simulink model "template_examples"  (R2024b)
settings: Solver=FixedStepDiscrete  StartTime=0.0  StopTime=10.0  RelTol=1e-3
libraries: hdlsllib x25, simulink x2
settings Model: Creator=foregan  LastModifiedBy=foregan
settings OptimizationCC: BlockReduction=off  ConditionallyExecuteInputs=off  DefaultParameterBehavior=Inlined
settings DebuggingCC: AlgebraicLoopMsg=error  SingleTaskRateTransMsg=error
settings RTWCC: GPUComputeCapability=3.5

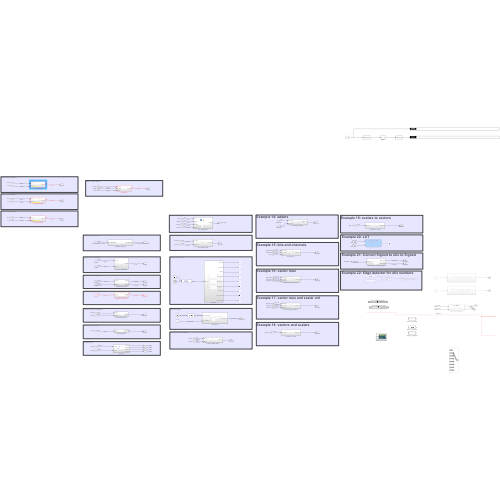
[thumbnail: Simulink's stored preview of the top-level diagram]
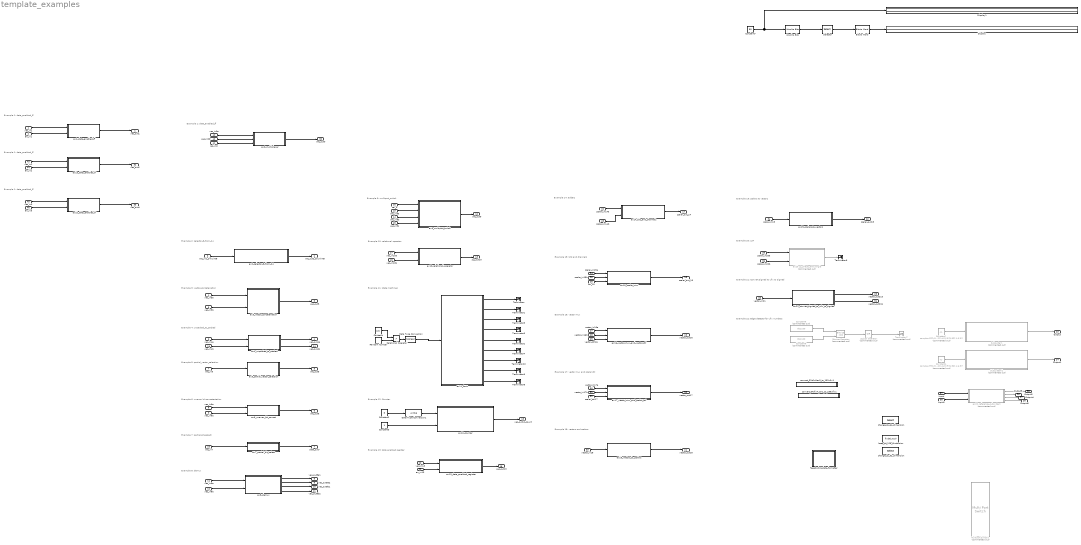
== system template_examples ==
  note: Example 22: Edge detector for ufix numbers
  note: Example 20: LUT
  note: Example 15: bits and channels
  note: Example 13: data enabled register
  note: Example 12: Counter
  note: Example 11: state machines
  note: Example 6: uneven bit concatentation
  note: Example 4: unpacked_to_packed
  note: Example 5: partial_vector_selection
  note: Example 3: vector_concatenation
  note: Example 2: selector_8_from_24
  note: Example 1: data_enabled_ff
  note: Example 7: partial_bit_select
  note: Example 8: demux
  note: Example 10: relational operator
  note: Example 9: multiport_switch
  note: Example 14: adders
  note: Example 16: vector mux
  note: Example 17: vector mux and scalar ctrl
  note: Example 18: vectors and scalars
  note: Example 19: scalars to vectors
  note: Example 21: Convert Signed to ufix to Signed
  note: Example 1: data_enabled_ff
  note: Example 1: data_enabled_ff
  note: Example 1: data_enabled_ff
  vec_in1 : Inport
  en_in1 : Inport  Port=2
  vec_in2_24xuint8 : Inport  Port=3  OutDataTypeStr=uint8  PortDimensions=24
  vec_in3a : Inport  Port=4  OutDataTypeStr=uint8  PortDimensions=2
  vec_in3b : Inport  Port=5  OutDataTypeStr=uint8  PortDimensions=2
  vec_in4a : Inport  Port=6  OutDataTypeStr=uint8  PortDimensions=4
  vec_in5 : Inport  Port=7  OutDataTypeStr=uint16
  vec_in6a : Inport  Port=8  OutDataTypeStr=fixdt(0,13,0)
  vec_in6b : Inport  Port=9  OutDataTypeStr=fixdt(0,5,0)
  vec_in7 : Inport  Port=10  OutDataTypeStr=fixdt(0,13,0)
  vec_in8a : Inport  Port=11  OutDataTypeStr=uint8  PortDimensions=[2 1]
  vec_in8b : Inport  Port=12  OutDataTypeStr=uint8  PortDimensions=2
  vec_in9a : Inport  Port=13  OutDataTypeStr=uint8
  vec_in9b : Inport  Port=14  OutDataTypeStr=uint8
  vec_in9c : Inport  Port=15  OutDataTypeStr=uint8
  sel_9 : Inport  Port=16  OutDataTypeStr=fixdt(0,2,0)
  vec_in10a : Inport  Port=17  OutDataTypeStr=int8
  vec_in10b : Inport  Port=18  OutDataTypeStr=int8
  vec_in4b : Inport  Port=19  OutDataTypeStr=uint8  PortDimensions=4
  vec_in13 : Inport  Port=20  OutDataTypeStr=fixdt(0,4,0)
  en_in13 : Inport  Port=21  OutDataTypeStr=boolean
  scalar_in14a : Inport  Port=22  OutDataTypeStr=fixdt(0,16,0)
  scalar_in14b : Inport  Port=23  OutDataTypeStr=fixdt(0,1,0)
  scalar_in15a : Inport  Port=24  OutDataTypeStr=fixdt(0,16,0)
  scalar_in15b : Inport  Port=25  OutDataTypeStr=fixdt(0,16,0)
  en_15 : Inport  Port=26  OutDataTypeStr=boolean
  vector_in16a : Inport  Port=27  OutDataTypeStr=fixdt(0,1,0)  PortDimensions=16
  vector_in16b : Inport  Port=28  OutDataTypeStr=fixdt(0,1,0)  PortDimensions=16
  vector_ctrl16 : Inport  Port=29  OutDataTypeStr=boolean  PortDimensions=16
  vector_in17a : Inport  Port=30  OutDataTypeStr=fixdt(0,1,0)  PortDimensions=16
  vector_in17b : Inport  Port=31  OutDataTypeStr=fixdt(0,1,0)  PortDimensions=16
  scalar_ctrl17 : Inport  Port=32  OutDataTypeStr=boolean  PortDimensions=1
  vector_in18 : Inport  Port=33  OutDataTypeStr=fixdt(0,1,0)  PortDimensions=16
  scalar_in19 : Inport  Port=34  OutDataTypeStr=fixdt(0,16,0)  PortDimensions=1
  scalar_in20a : Inport  Port=35  OutDataTypeStr=fixdt(1,4,0)
  scalar_in20b : Inport  Port=36  OutDataTypeStr=fixdt(1,4,0)
  Input : Inport  Port=37  OutDataTypeStr=boolean
  Input1 : Inport  Port=38  OutDataTypeStr=boolean
  vector_in21 : Inport  Port=39  OutDataTypeStr=fixdt(1,4,1)  PortDimensions=2
  vec_in0a : Inport  Port=40
  sel_in0 : Inport  Port=41
  vec_in0b : Inport  Port=42  OutDataTypeStr=uint8
  vec_in2 : Inport  Port=43
  en_in2 : Inport  Port=44
  vec_in3 : Inport  Port=45
  en_in3 : Inport  Port=46
  Bits to Word : hdlsllib/Logic and Bit Operations/Bits to Word  bitOrder=LSB first  signedOutputValues=Unsigned
  Bitwise Operator : simulink/Logic and Bit Operations/Bitwise Operator  Commented=on  logicop=XOR  UseBitMask=off  NumInputPorts=2  BitMask=bin2dec('11011001')  BitMaskRealWorld=Stored Integer
  Constant : Constant  Value=0.5  SampleTime=1
  Constant1 : Constant  Commented=on  Value=complex(fi([1:32],1,6,3),fi([1:32],1,6,3))'  OutDataTypeStr=fixdt(1,6,3)
  Constant2 : Constant  Value=5
  Constant3 : Constant  OutDataTypeStr=boolean
  Constant4 : Constant  Commented=on  Value=complex(fi([1:32],1,6,3),fi([1:32],1,6,3))'  OutDataTypeStr=fixdt(1,6,3)
  Constant5 : Constant  Commented=on  Value=0b1100  OutDataTypeStr=fixdt(0,4,0)  SampleTime=1
  Constant6 : Constant  Commented=on  Value=0b1100  OutDataTypeStr=fixdt(0,4,0)  SampleTime=1
  Constant7 : Constant  Value=55  OutDataTypeStr=fixdt(0,128,0)  SampleTime=1
  Data Type Conversion : DataTypeConversion  OutDataTypeStr=boolean  SaturateOnIntegerOverflow=off  RndMeth=Floor
  Data Type Conversion1 : DataTypeConversion  OutDataTypeStr=uint16  SaturateOnIntegerOverflow=off  RndMeth=Floor
  Display : Display
      settings: Format=binary (Stored Integer)
  Display1 : Display
      settings: Format=binary (Stored Integer)
  Logical Operator : Logic  Commented=on  Operator=OR  Inputs=1  AllPortsSameDT=off  OutDataTypeStr=boolean
  Multiport Switch1 : MultiPortSwitch  Commented=on  DataPortOrder=Zero-based contiguous  Inputs=7  zeroidx=on  SaturateOnIntegerOverflow=off  InputSameDT=off
  Random Number : RandomNumber  SampleTime=1
  Relational Operator : RelationalOperator  Operator=>  OutDataTypeStr=boolean  RndMeth=Simplest  InputSameDT=off
  Selector : Selector  IndexMode=Zero-based  InputPortWidth=128  IndexOptions=Index vector (dialog)  Indices=[127:-1:0]  OutputSizes=1
  Subsystem : Subsystem  Commented=on
  Subsystem1 : Subsystem  Commented=on
  Terminator{,1..6,8..10} (10 alike) : Terminator
  Terminator7 : Terminator  Commented=on
  Word to Bits : hdlsllib/Logic and Bit Operations/Word to Bits  maxWordLength=128  bitOrder=LSB first
  change_to_32_dimension : Selector  InputPortWidth=128  IndexOptions=Index vector (dialog)  Indices=[1:32]  OutputSizes=1
  change_to_64_dimension : Selector  InputPortWidth=128  IndexOptions=Index vector (dialog)  Indices=[1:64]  OutputSizes=1
  convert_32sfix6en3_to_192ufix1 : Subsystem  TreatAsAtomicUnit=on
  convert_64sfix4_en1_to_256ufix1 : Subsystem  TreatAsAtomicUnit=on
  ex0_multiplexer : Subsystem
  ex10_relational_operator : Subsystem
  ex11_fsms : Subsystem
  ex12_counter : Subsystem
  ex13_data_enabled_register : Subsystem
  ex14_bits_and_channels : Subsystem
  ex15_scalar_mux : Subsystem
  ex16_vector_mux_and_vector_ctrl : Subsystem
  ex17_vector_mux_and_scalar_ctrl : Subsystem
  ex18_vectors_to_scalars : Subsystem
  ex19_scalars_to_vectors : Subsystem
  ex1_data_enabled_ff : Subsystem
  ex1a_data_enabled_ff : Subsystem
  ex1b_data_enabled_ff : Subsystem
  ex20_cs_phase_error_angle : Subsystem  Tag=DecoupledSystem  Commented=on  ReferencedSubsystem=cs_phase_error_angle
  ex21_convert_signed_to_ufix_to_signed : Subsystem
  ex22_reference_subsystem : Subsystem  Commented=on
  ex2_selector_8_from_24 : Subsystem
  ex3_vector_concatenation : Subsystem
  ex4_unpacked_to_packed : Subsystem
  ex5_partial_vector_selection : Subsystem
  ex6_uneven_bit_concat : Subsystem
  ex7_partial_bit_select : Subsystem
  ex8_demux : Subsystem
  ex9_multiport_switch : Subsystem
  fpga2odwt_data_formatter : Subsystem
  keep_at_128_dimension : DataTypeConversion  OutDataTypeStr=fixdt(1,6,3)  SaturateOnIntegerOverflow=off  RndMeth=Floor
  vec_out1 : Outport
  vec_out2_8xunint8 : Outport  Port=2
  vec_out3 : Outport  Port=3
  vec_out4a : Outport  Port=4
  vec_out5 : Outport  Port=5  OutDataTypeStr=uint8
  vec_out6 : Outport  Port=6  OutDataTypeStr=fixdt(0,18,0)
  data_out7 : Outport  Port=7  OutDataTypeStr=fixdt(0,1,0)
  vec_out8a1 : Outport  Port=8
  vec_out8a2 : Outport  Port=9
  vec_out8b1 : Outport  Port=10
  vec_out8b2 : Outport  Port=11
  vec_out9 : Outport  Port=12  OutDataTypeStr=uint8
  sig_out10 : Outport  Port=13
  vec_out4b : Outport  Port=14
  vec_out12_count : Outport  Port=15
  vec_out13 : Outport  Port=16
  scalar_out_14 : Outport  Port=17
  "scalar_out_15 " : Outport  Port=18
  vector_out16 : Outport  Port=19  PortDimensions=16
  vector_out17 : Outport  Port=20  PortDimensions=16
  vector_out18 : Outport  Port=21
  scalar_out19 : Outport  Port=22  PortDimensions=16
  Output : Outport  Port=23
  Output1 : Outport  Port=24
  Output2 : Outport  Port=25
  Output3 : Outport  Port=26
  Output4 : Outport  Port=27
  Output5 : Outport  Port=28
  vector_out21a : Outport  Port=29
  vec_out0 : Outport  Port=30
  vector_out21b : Outport  Port=31
  vec_out2 : Outport  Port=32
  vec_out4 : Outport  Port=33
  wires:
  vec_in1/1 -> ex1_data_enabled_ff/1(vec_in1)  "data_in1"
  en_in1/1 -> ex1_data_enabled_ff/2(en_in1)  "enable1"
  ex1_data_enabled_ff/1(vec_out1) -> vec_out1/1  "vec_out1"
  vec_in2_24xuint8/1 -> ex2_selector_8_from_24/1(vec_in2_24xuint8)  "vec_in2_24xuint8"
  ex2_selector_8_from_24/1(vec_out2_8xunint8) -> vec_out2_8xunint8/1  "vec_out2_8xunint8"
  vec_in3a/1 -> ex3_vector_concatenation/1(vec_in3a)  "vec_in3a"
  vec_in3b/1 -> ex3_vector_concatenation/2(vec_in3b)  "vec_in3b"
  ex3_vector_concatenation/1(vec_out3) -> vec_out3/1  "vec_out3"
  vec_in4a/1 -> ex4_unpacked_to_packed/1(vec_in4a)  "vec_in4a"
  ex4_unpacked_to_packed/1(vec_out4a) -> vec_out4a/1  "vec_out4a"
  vec_in5/1 -> ex5_partial_vector_selection/1(vec_in5)  "vec_in5"
  ex5_partial_vector_selection/1(vec_out5) -> vec_out5/1  "vec_out5"
  vec_in6a/1 -> ex6_uneven_bit_concat/1(vec_in6a)
  vec_in6b/1 -> ex6_uneven_bit_concat/2(vec_in6b)
  ex6_uneven_bit_concat/1(vec_out6) -> vec_out6/1
  vec_in7/1 -> ex7_partial_bit_select/1(vec_in7)  "vec_in7"
  ex7_partial_bit_select/1(data_out7) -> data_out7/1
  ex8_demux/4(vec_out8b2) -> vec_out8b2/1
  ex8_demux/3(vec_out8b1) -> vec_out8b1/1
  vec_in8b/1 -> ex8_demux/2(vec_in8b)
  ex8_demux/2(vec_out8a2) -> vec_out8a2/1
  ex8_demux/1(vec_out8a1) -> vec_out8a1/1
  vec_in8a/1 -> ex8_demux/1(vec_in8a)
  sel_9/1 -> ex9_multiport_switch/1(sel_9)  "sel_9"
  vec_in9a/1 -> ex9_multiport_switch/2(vec_in9a)  "vec_in9a"
  vec_in9b/1 -> ex9_multiport_switch/3(vec_in9b)  "vec_in9b"
  vec_in9c/1 -> ex9_multiport_switch/4(vec_in9c)  "vec_in9c"
  ex9_multiport_switch/1(vec_out9) -> vec_out9/1
  vec_in10a/1 -> ex10_relational_operator/1(vec_in10a)  "vec_in10a"
  vec_in10b/1 -> ex10_relational_operator/2(vec_in10b)  "vec_in10b"
  ex10_relational_operator/1(sig_out10) -> sig_out10/1
  ex4_unpacked_to_packed/2(vec_out4b) -> vec_out4b/1  "vec_out4b"
  vec_in4b/1 -> ex4_unpacked_to_packed/2(vec_in4b)  "vec_in4b"
  Relational Operator/1 -> Data Type Conversion/1
  Random Number/1 -> Relational Operator/2
  Constant/1 -> Relational Operator/1
  Constant2/1 -> Data Type Conversion1/1  "vec_in12_count_to"
  Constant3/1 -> ex12_counter/2(sel_in12_enable)  "sel_in12_enable"
  ex12_counter/1(vec_out12_count) -> vec_out12_count/1  "vec_out12_count"
  Data Type Conversion1/1 -> ex12_counter/1(vec_in12_count_to)  "vec_in12_count_to"
  vec_in13/1 -> ex13_data_enabled_register/1(data_in13)  "data_in13"
  en_in13/1 -> ex13_data_enabled_register/2(enable13)  "enable13"
  ex13_data_enabled_register/1(vec_out13) -> vec_out13/1
  Data Type Conversion/1 -> ex11_fsms/1(sel11a)  "sel11a"
  ex11_fsms/1(mf_out11a) -> Terminator/1
  ex11_fsms/2(mf_out11b) -> Terminator1/1
  ex11_fsms/3(mf_state) -> Terminator3/1
  ex11_fsms/4(dum_sf_state) -> Terminator5/1
  ex11_fsms/5(dum_sf_out11a) -> Terminator2/1
  ex11_fsms/6(dum_sf_out11b) -> Terminator4/1
  scalar_in14a/1 -> ex14_bits_and_channels/1(scalar_in14a)
  scalar_in14b/1 -> ex14_bits_and_channels/2(scalar_in14b)
  ex14_bits_and_channels/1(scalar_out_14) -> scalar_out_14/1
  ex15_scalar_mux/1(scalar_out_15) -> "scalar_out_15 "/1
  scalar_in15b/1 -> ex15_scalar_mux/2(scalar_in15b)
  scalar_in15a/1 -> ex15_scalar_mux/1(scalar_in15a)
  en_15/1 -> ex15_scalar_mux/3(en_15)
  vector_ctrl16/1 -> ex16_vector_mux_and_vector_ctrl/3(vector_ctrl16)
  vector_in16b/1 -> ex16_vector_mux_and_vector_ctrl/2(vector_in16b)
  vector_in16a/1 -> ex16_vector_mux_and_vector_ctrl/1(vector_in16a)
  ex16_vector_mux_and_vector_ctrl/1(vector_out16) -> vector_out16/1
  vector_in17b/1 -> ex17_vector_mux_and_scalar_ctrl/2(vector_in17b)
  scalar_ctrl17/1 -> ex17_vector_mux_and_scalar_ctrl/3(scalar_ctrl17)
  vector_in17a/1 -> ex17_vector_mux_and_scalar_ctrl/1(vector_in17a)
  ex17_vector_mux_and_scalar_ctrl/1(scalar_out_17) -> vector_out17/1
  vector_in18/1 -> ex18_vectors_to_scalars/1(vector_in18)
  ex18_vectors_to_scalars/1(scalar_out_18) -> vector_out18/1
  ex19_scalars_to_vectors/1(scalar_out19) -> scalar_out19/1
  scalar_in19/1 -> ex19_scalars_to_vectors/1(scalar_in19)
  scalar_in20a/1 -> ex20_cs_phase_error_angle/1
  scalar_in20b/1 -> ex20_cs_phase_error_angle/2
  ex20_cs_phase_error_angle/1 -> Terminator6/1
  Constant1/1 -> Subsystem/1(In1)
  Subsystem/1(y) -> Output/1
  Subsystem1/1(y) -> Output1/1
  Constant4/1 -> Subsystem1/1(In1)
  Input/1 -> ex22_reference_subsystem/1(In1)
  ex22_reference_subsystem/1(Out1) -> Output2/1
  ex22_reference_subsystem/2(Output3) -> Output3/1
  ex22_reference_subsystem/3(Output) -> Output4/1
  ex22_reference_subsystem/4(Output1) -> Output5/1
  Input1/1 -> ex22_reference_subsystem/2(Input1)
  ex0_multiplexer/1(vec_out0) -> vec_out0/1  "vec_out0"
  sel_in0/1 -> ex0_multiplexer/3(sel_in0)  "sel_in0"
  vec_in0a/1 -> ex0_multiplexer/1(vec_in0a)  "vec_in0a"
  vec_in0b/1 -> ex0_multiplexer/2(vec_in0b)  "vec_in0b"
  vector_in21/1 -> ex21_convert_signed_to_ufix_to_signed/1(vector_in21)  "vector_in21"
  ex21_convert_signed_to_ufix_to_signed/1(vector_out21a) -> vector_out21a/1  "vector_out21a"
  ex21_convert_signed_to_ufix_to_signed/2(vector_out21b) -> vector_out21b/1  "vector_out21b"
  Bitwise Operator/1 -> Logical Operator/1
  Constant6/1 -> Bitwise Operator/2
  Logical Operator/1 -> Terminator7/1  "has_peak_count_changed"
  Constant5/1 -> Bitwise Operator/1
  Word to Bits/1 -> Selector/1
  Constant7/1 -> Display1/1, Word to Bits/1
  Selector/1 -> Bits to Word/1
  Bits to Word/1 -> Display/1
  ex11_fsms/7(ium_sf_state) -> Terminator10/1
  ex11_fsms/8(ium_sm_out11a) -> Terminator9/1
  ex11_fsms/9(ium_sm_out11b) -> Terminator8/1
  ex1a_data_enabled_ff/1(vec_out1) -> vec_out2/1  "vec_out1"
  en_in2/1 -> ex1a_data_enabled_ff/2(en_in1)  "enable1"
  vec_in2/1 -> ex1a_data_enabled_ff/1(vec_in1)  "data_in1"
  ex1b_data_enabled_ff/1(vec_out1) -> vec_out4/1  "vec_out1"
  vec_in3/1 -> ex1b_data_enabled_ff/1(vec_in1)  "data_in1"
  en_in3/1 -> ex1b_data_enabled_ff/2(en_in1)  "enable1"
  ? -> ?  "<path_select>"

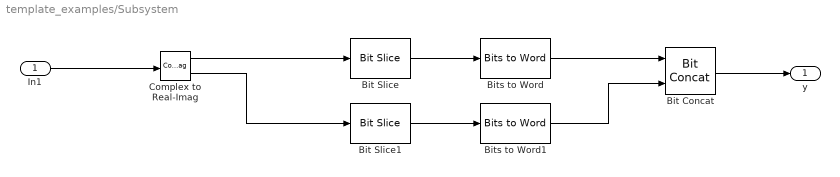
== system template_examples/Subsystem ==
  In1 : Inport
  Bit Concat : hdlsllib/Logic and Bit Operations/Bit Concat  numInputs=2
  Bit Slice : hdlsllib/Logic and Bit Operations/Bit Slice  lidx=4  ridx=4
  Bit Slice1 : hdlsllib/Logic and Bit Operations/Bit Slice  lidx=4  ridx=4
  Bits to Word : hdlsllib/Logic and Bit Operations/Bits to Word
  Bits to Word1 : hdlsllib/Logic and Bit Operations/Bits to Word
  Complex to Real-Imag : ComplexToRealImag
  y : Outport
  wires:
  Bit Slice/1 -> Bits to Word/1
  Bits to Word/1 -> Bit Concat/1
  Complex to Real-Imag/1 -> Bit Slice/1
  Bit Concat/1 -> y/1
  Bit Slice1/1 -> Bits to Word1/1
  In1/1 -> Complex to Real-Imag/1
  Bits to Word1/1 -> Bit Concat/2
  Complex to Real-Imag/2 -> Bit Slice1/1

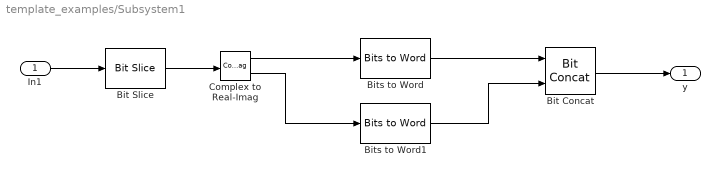
== system template_examples/Subsystem1 ==
  In1 : Inport
  Bit Concat : hdlsllib/Logic and Bit Operations/Bit Concat  numInputs=2
  Bit Slice : hdlsllib/Logic and Bit Operations/Bit Slice  lidx=4  ridx=4
  Bits to Word : hdlsllib/Logic and Bit Operations/Bits to Word
  Bits to Word1 : hdlsllib/Logic and Bit Operations/Bits to Word
  Complex to Real-Imag : ComplexToRealImag
  y : Outport
  wires:
  Complex to Real-Imag/1 -> Bits to Word/1
  Bits to Word/1 -> Bit Concat/1
  Bit Concat/1 -> y/1
  Complex to Real-Imag/2 -> Bits to Word1/1
  In1/1 -> Bit Slice/1
  Bits to Word1/1 -> Bit Concat/2
  Bit Slice/1 -> Complex to Real-Imag/1

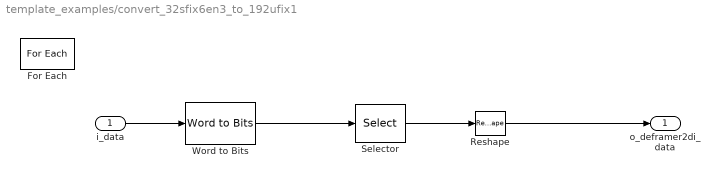
== system template_examples/convert_32sfix6en3_to_192ufix1 ==
  i_data : Inport  Partition=on  PartitionDimension=1  PartitionWidth=1  PartitionOffset=0
  For Each : ForEach  DisableCoverage=on
  Reshape : Reshape
  Selector : Selector  InputPortWidth=6  IndexOptions=Index vector (dialog)  Indices=[1:6]  OutputSizes=1
  Word to Bits : hdlsllib/Logic and Bit Operations/Word to Bits  maxWordLength=6  bitOrder=LSB first
  o_deframer2di_data : Outport  ConcatenationDimension=1
  wires:
  i_data/1 -> Word to Bits/1
  Word to Bits/1 -> Selector/1
  Selector/1 -> Reshape/1
  Reshape/1 -> o_deframer2di_data/1

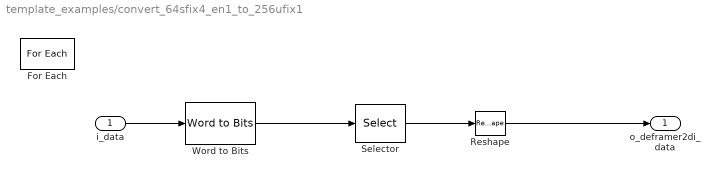
== system template_examples/convert_64sfix4_en1_to_256ufix1 ==
  i_data : Inport  Partition=on  PartitionDimension=1  PartitionWidth=1  PartitionOffset=0
  For Each : ForEach  DisableCoverage=on
  Reshape : Reshape
  Selector : Selector  InputPortWidth=4  IndexOptions=Index vector (dialog)  Indices=[1:4]  OutputSizes=1
  Word to Bits : hdlsllib/Logic and Bit Operations/Word to Bits  maxWordLength=4  bitOrder=LSB first
  o_deframer2di_data : Outport  ConcatenationDimension=1
  wires:
  i_data/1 -> Word to Bits/1
  Word to Bits/1 -> Selector/1
  Selector/1 -> Reshape/1
  Reshape/1 -> o_deframer2di_data/1

== system template_examples/ex0_multiplexer ==
  vec_in0a : Inport  OutDataTypeStr=uint8
  vec_in0b : Inport  Port=2
  sel_in0 : Inport  Port=3  OutDataTypeStr=boolean
  enable_mux : Switch  Criteria=u2 ~= 0  Threshold=1  OutDataTypeStr=uint8  ZeroCross=off  SaturateOnIntegerOverflow=off  InputSameDT=off
  vec_out0 : Outport  OutDataTypeStr=uint8
  wires:
  sel_in0/1 -> enable_mux/2  "en_in1"
  enable_mux/1 -> vec_out0/1  "mux_out"
  vec_in0a/1 -> enable_mux/1  "vec_in1"
  vec_in0b/1 -> enable_mux/3  "vec_in0b"

== system template_examples/ex10_relational_operator ==
  vec_in10a : Inport
  vec_in10b : Inport  Port=2
  Relational Operator : RelationalOperator  Operator=>  OutDataTypeStr=boolean  RndMeth=Simplest  InputSameDT=off
  sig_out10 : Outport
  wires:
  vec_in10a/1 -> Relational Operator/1
  vec_in10b/1 -> Relational Operator/2
  Relational Operator/1 -> sig_out10/1  "sig_out10"

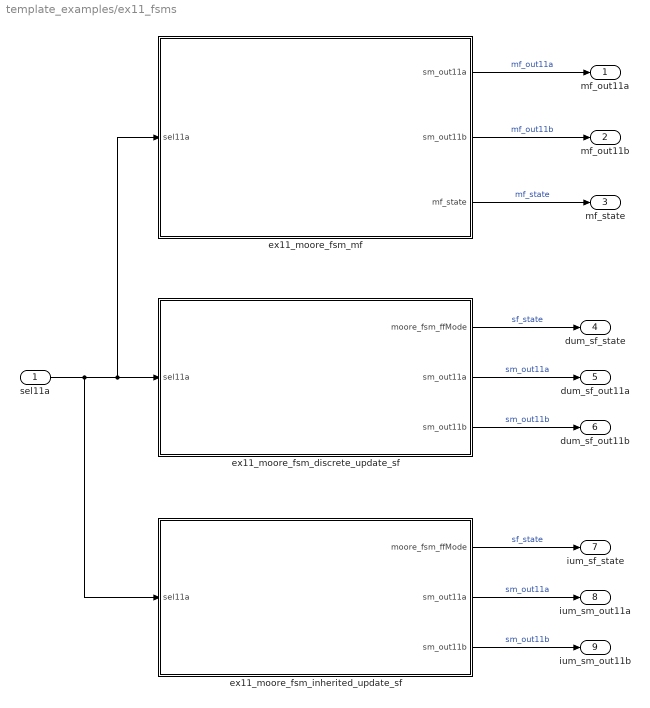
== system template_examples/ex11_fsms ==
  sel11a : Inport
  ex11_moore_fsm_discrete_update_sf : Stateflow chart  TreatAsAtomicUnit=on
  ex11_moore_fsm_inherited_update_sf : Stateflow chart  TreatAsAtomicUnit=on
  ex11_moore_fsm_mf : MATLAB Function  TreatAsAtomicUnit=on
  mf_out11a : Outport
  mf_out11b : Outport  Port=2
  mf_state : Outport  Port=3
  dum_sf_state : Outport  Port=4
  dum_sf_out11a : Outport  Port=5
  dum_sf_out11b : Outport  Port=6
  ium_sf_state : Outport  Port=7
  ium_sm_out11a : Outport  Port=8
  ium_sm_out11b : Outport  Port=9
  wires:
  ex11_moore_fsm_discrete_update_sf/2(sm_out11a) -> dum_sf_out11a/1  "sm_out11a"
  ex11_moore_fsm_mf/1(sm_out11a) -> mf_out11a/1  "mf_out11a"
  ex11_moore_fsm_mf/2(sm_out11b) -> mf_out11b/1  "mf_out11b"
  ex11_moore_fsm_mf/3(mf_state) -> mf_state/1  "mf_state"
  ex11_moore_fsm_discrete_update_sf/3(sm_out11b) -> dum_sf_out11b/1  "sm_out11b"
  ex11_moore_fsm_discrete_update_sf/1(moore_fsm_ffMode) -> dum_sf_state/1  "sf_state"
  ex11_moore_fsm_inherited_update_sf/3(sm_out11b) -> ium_sm_out11b/1  "sm_out11b"
  ex11_moore_fsm_inherited_update_sf/2(sm_out11a) -> ium_sm_out11a/1  "sm_out11a"
  ex11_moore_fsm_inherited_update_sf/1(moore_fsm_ffMode) -> ium_sf_state/1  "sf_state"
  sel11a/1 -> ex11_moore_fsm_inherited_update_sf/1(sel11a), ex11_moore_fsm_mf/1(sel11a), ex11_moore_fsm_discrete_update_sf/1(sel11a)

== system template_examples/ex12_counter ==
  vec_in12_count_to : Inport
  sel_in12_enable : Inport  Port=2
  Relational Operator1 : RelationalOperator  Operator===  OutDataTypeStr=boolean  RndMeth=Simplest  InputSameDT=off
  example_12_16b_counter : hdlsllib/Sources/HDL Counter  CountType=Count limited  CountInit=0  CountStep=1  CountMax=25  CountFromType=Initial value  CountFrom=0  CountResetPort=on  CountLoadPort=off  CountEnbPort=on  CountDirPort=off  CountHitOutputPort=off  CountDataType=Unsigned  CountWordLen=16  CountFracLen=0  CountSampTime=1
  vec_out12_count : Outport
  wires:
  Relational Operator1/1 -> example_12_16b_counter/1
  example_12_16b_counter/1 -> vec_out12_count/1, Relational Operator1/2  "vec_out12_count"
  vec_in12_count_to/1 -> Relational Operator1/1
  sel_in12_enable/1 -> example_12_16b_counter/2

== system template_examples/ex13_data_enabled_register ==
  data_in13 : Inport
  enable13 : Inport  Port=2
  Unit Delay Enabled Synchronous : hdlsllib/Discrete/Unit Delay Enabled Synchronous  InitialCondition=0.0  SampleTime=-1
  vec_out13 : Outport
  wires:
  Unit Delay Enabled Synchronous/1 -> vec_out13/1  "vec_out13"
  data_in13/1 -> Unit Delay Enabled Synchronous/1
  enable13/1 -> Unit Delay Enabled Synchronous/2

== system template_examples/ex14_bits_and_channels ==
  scalar_in14a : Inport
  scalar_in14b : Inport  Port=2
  Add : Sum  OutDataTypeStr=Inherit: Keep MSB
  scalar_out_14 : Outport
  wires:
  Add/1 -> scalar_out_14/1  "scalar_out_14"
  scalar_in14b/1 -> Add/2  "scalar_in14b"
  scalar_in14a/1 -> Add/1  "scalar_in14a"

== system template_examples/ex15_scalar_mux ==
  scalar_in15a : Inport
  scalar_in15b : Inport  Port=2
  en_15 : Inport  Port=3
  Switch : Switch  Criteria=u2 ~= 0  SaturateOnIntegerOverflow=off  InputSameDT=off
  scalar_out_15 : Outport
  wires:
  Switch/1 -> scalar_out_15/1  "scalar_out_15"
  scalar_in15b/1 -> Switch/3  "scalar_in15b"
  scalar_in15a/1 -> Switch/1  "scalar_in15a"
  en_15/1 -> Switch/2

== system template_examples/ex16_vector_mux_and_vector_ctrl ==
  vector_in16a : Inport
  vector_in16b : Inport  Port=2
  vector_ctrl16 : Inport  Port=3
  Switch : Switch  Criteria=u2 ~= 0  SaturateOnIntegerOverflow=off  InputSameDT=off
  vector_out16 : Outport
  wires:
  Switch/1 -> vector_out16/1  "scalar_out_16"
  vector_in16b/1 -> Switch/3  "vector_in16b"
  vector_in16a/1 -> Switch/1  "vector_in16a"
  vector_ctrl16/1 -> Switch/2  "vector_ctrl16"

== system template_examples/ex17_vector_mux_and_scalar_ctrl ==
  vector_in17a : Inport
  vector_in17b : Inport  Port=2
  scalar_ctrl17 : Inport  Port=3
  Switch : Switch  Criteria=u2 ~= 0  SaturateOnIntegerOverflow=off  InputSameDT=off
  scalar_out_17 : Outport
  wires:
  Switch/1 -> scalar_out_17/1  "scalar_out_17"
  vector_in17b/1 -> Switch/3  "vector_in17b"
  vector_in17a/1 -> Switch/1  "vector_in17a"
  scalar_ctrl17/1 -> Switch/2  "scalar_ctrl17"

== system template_examples/ex18_vectors_to_scalars ==
  vector_in18 : Inport
  Bits to Word : hdlsllib/Logic and Bit Operations/Bits to Word  bitOrder=LSB first  signedOutputValues=Unsigned
  Data Type Conversion : DataTypeConversion  OutDataTypeStr=fixdt(0,1,0)  SaturateOnIntegerOverflow=off  RndMeth=Floor
  Logical Operator : Logic  Operator=NOT  IconShape=distinctive  AllPortsSameDT=off  OutDataTypeStr=boolean
  scalar_out_18 : Outport
  wires:
  Logical Operator/1 -> Data Type Conversion/1  "scalar_out_18"
  vector_in18/1 -> Logical Operator/1  "vector_in18a"
  Bits to Word/1 -> scalar_out_18/1
  Data Type Conversion/1 -> Bits to Word/1

== system template_examples/ex19_scalars_to_vectors ==
  scalar_in19 : Inport
  Logical Operator : Logic  Operator=NOT  IconShape=distinctive  AllPortsSameDT=off  OutDataTypeStr=boolean
  Word to Bits : hdlsllib/Logic and Bit Operations/Word to Bits  maxWordLength=16  bitOrder=LSB first
  scalar_out19 : Outport
  wires:
  scalar_in19/1 -> Word to Bits/1  "scalar_in19"
  Logical Operator/1 -> scalar_out19/1  "scalar_out19"
  Word to Bits/1 -> Logical Operator/1

== system template_examples/ex1_data_enabled_ff ==
  note: mux_out = enable ? vec_in1 : vec_out1
  vec_in1 : Inport  OutDataTypeStr=uint8
  en_in1 : Inport  Port=2  OutDataTypeStr=boolean
  Delay : Delay  DelayLength=1
  enable_mux : Switch  Criteria=u2 ~= 0  Threshold=1  OutDataTypeStr=uint8  ZeroCross=off  SaturateOnIntegerOverflow=off  InputSameDT=off
  vec_out1 : Outport  OutDataTypeStr=uint8
  wires:
  Delay/1 -> enable_mux/3, vec_out1/1  "vec_out1"
  en_in1/1 -> enable_mux/2  "en_in1"
  enable_mux/1 -> Delay/1  "mux_out"
  vec_in1/1 -> enable_mux/1  "vec_in1"

== system template_examples/ex1a_data_enabled_ff ==
  note: mux_out = enable ? vec_in1 : vec_out1
  vec_in1 : Inport  OutDataTypeStr=uint8
  en_in1 : Inport  Port=2  OutDataTypeStr=boolean
  Unit Delay Enabled Synchronous : hdlsllib/Discrete/Unit Delay Enabled Synchronous  InitialCondition=0.0  SampleTime=-1
  vec_out1 : Outport  OutDataTypeStr=uint8
  wires:
  Unit Delay Enabled Synchronous/1 -> vec_out1/1  "vec_out1"
  en_in1/1 -> Unit Delay Enabled Synchronous/2  "en_in1"
  vec_in1/1 -> Unit Delay Enabled Synchronous/1  "vec_in1"

== system template_examples/ex1b_data_enabled_ff ==
  note: mux_out = enable ? vec_in1 : vec_out1
  vec_in1 : Inport  OutDataTypeStr=uint8
  en_in1 : Inport  Port=2  OutDataTypeStr=boolean
  MATLAB Function : MATLAB Function  TreatAsAtomicUnit=on
  vec_out1 : Outport  OutDataTypeStr=uint8
  wires:
  MATLAB Function/1(y) -> vec_out1/1  "vec_out1"
  en_in1/1 -> MATLAB Function/2(u)  "en_in1"
  vec_in1/1 -> MATLAB Function/1(vec_in1)  "vec_in1"

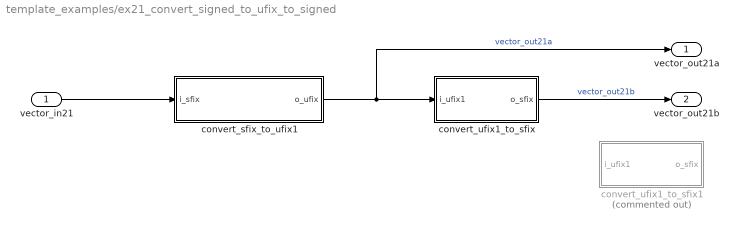
== system template_examples/ex21_convert_signed_to_ufix_to_signed ==
  vector_in21 : Inport
  convert_sfix_to_ufix1 : Subsystem  TreatAsAtomicUnit=on
  convert_ufix1_to_sfix : Subsystem  TreatAsAtomicUnit=on
  convert_ufix1_to_sfix1 : Subsystem  Commented=on  TreatAsAtomicUnit=on
  vector_out21a : Outport
  vector_out21b : Outport  Port=2
  wires:
  convert_sfix_to_ufix1/1(o_ufix) -> convert_ufix1_to_sfix/1(i_ufix1), vector_out21a/1  "vector_out21a"
  vector_in21/1 -> convert_sfix_to_ufix1/1(i_sfix)
  convert_ufix1_to_sfix/1(o_sfix) -> vector_out21b/1  "vector_out21b"

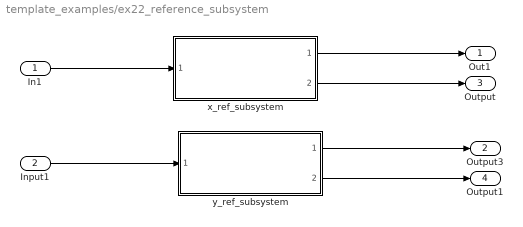
== system template_examples/ex22_reference_subsystem ==
  In1 : Inport
  Input1 : Inport  Port=2
  x_ref_subsystem : Subsystem  ReferencedSubsystem=example_ref_subsystem
  y_ref_subsystem : Subsystem  ReferencedSubsystem=example_ref_subsystem
  Out1 : Outport
  Output3 : Outport  Port=2
  Output : Outport  Port=3
  Output1 : Outport  Port=4
  wires:
  y_ref_subsystem/1 -> Output3/1
  Input1/1 -> y_ref_subsystem/1
  In1/1 -> x_ref_subsystem/1
  x_ref_subsystem/1 -> Out1/1
  x_ref_subsystem/2 -> Output/1
  y_ref_subsystem/2 -> Output1/1

== system template_examples/ex2_selector_8_from_24 ==
  vec_in2_24xuint8 : Inport
  select_lower_8 : Selector  InputPortWidth=24  IndexOptions=Index vector (dialog)  Indices=[1:8]  OutputSizes=1
  vec_out2_8xunint8 : Outport
  wires:
  select_lower_8/1 -> vec_out2_8xunint8/1  "vec_out2_8xunint8"
  vec_in2_24xuint8/1 -> select_lower_8/1

== system template_examples/ex3_vector_concatenation ==
  vec_in3a : Inport
  vec_in3b : Inport  Port=2
  Vector Concatenate : Concatenate
  vec_out3 : Outport
  wires:
  vec_in3b/1 -> Vector Concatenate/2  "vec_in3b"
  Vector Concatenate/1 -> vec_out3/1  "vec_out3"
  vec_in3a/1 -> Vector Concatenate/1  "vec_in3a"

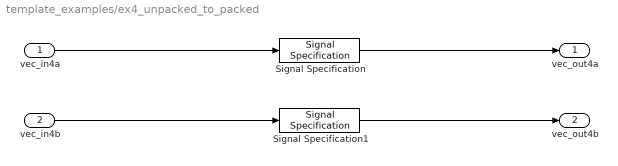
== system template_examples/ex4_unpacked_to_packed ==
  vec_in4a : Inport
  vec_in4b : Inport  Port=2  PortDimensions=4
  Signal Specification : SignalSpecification  OutDataTypeStr=uint8  Dimensions=[4 1]
  Signal Specification1 : SignalSpecification
  vec_out4a : Outport
  vec_out4b : Outport  Port=2  PortDimensions=4
  wires:
  Signal Specification/1 -> vec_out4a/1
  vec_in4a/1 -> Signal Specification/1
  vec_in4b/1 -> Signal Specification1/1
  Signal Specification1/1 -> vec_out4b/1

== system template_examples/ex5_partial_vector_selection ==
  vec_in5 : Inport
  select_8_lsbs : simulink/Logic and Bit Operations/Extract Bits  bitsToExtract=Range of bits  numBits=8  bitIdxRange=[0 7]  outScalingMode=Preserve fixed-point scaling
  vec_out5 : Outport  OutDataTypeStr=uint8
  wires:
  select_8_lsbs/1 -> vec_out5/1  "vec_out5"
  vec_in5/1 -> select_8_lsbs/1  "vec_in5"

== system template_examples/ex6_uneven_bit_concat ==
  vec_in6a : Inport
  vec_in6b : Inport  Port=2
  Bit Concat : hdlsllib/Logic and Bit Operations/Bit Concat  numInputs=2
  vec_out6 : Outport
  wires:
  vec_in6a/1 -> Bit Concat/1
  Bit Concat/1 -> vec_out6/1
  vec_in6b/1 -> Bit Concat/2

== system template_examples/ex7_partial_bit_select ==
  vec_in7 : Inport
  bit7 : hdlsllib/Logic and Bit Operations/Bit Slice  lidx=7  ridx=7
  data_out7 : Outport  OutDataTypeStr=fixdt(0,1,0)
  wires:
  vec_in7/1 -> bit7/1  "vec_in7"
  bit7/1 -> data_out7/1  "data_out7"

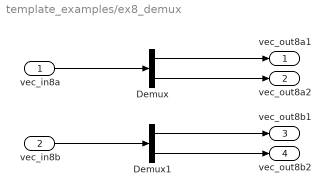
== system template_examples/ex8_demux ==
  vec_in8a : Inport
  vec_in8b : Inport  Port=2
  Demux : Demux  Outputs=2
  Demux1 : Demux  Outputs=2
  vec_out8a1 : Outport
  vec_out8a2 : Outport  Port=2
  vec_out8b1 : Outport  Port=3
  vec_out8b2 : Outport  Port=4
  wires:
  Demux1/1 -> vec_out8b1/1
  Demux/2 -> vec_out8a2/1
  Demux1/2 -> vec_out8b2/1
  Demux/1 -> vec_out8a1/1
  vec_in8b/1 -> Demux1/1
  vec_in8a/1 -> Demux/1

== system template_examples/ex9_multiport_switch ==
  sel_9 : Inport
  vec_in9a : Inport  Port=2
  vec_in9b : Inport  Port=3
  vec_in9c : Inport  Port=4
  Multiport Switch : MultiPortSwitch  DataPortOrder=Zero-based contiguous  zeroidx=on  SaturateOnIntegerOverflow=off  InputSameDT=off
  vec_out9 : Outport
  wires:
  Multiport Switch/1 -> vec_out9/1  "vec_out9"
  vec_in9c/1 -> Multiport Switch/4
  vec_in9a/1 -> Multiport Switch/2
  sel_9/1 -> Multiport Switch/1
  vec_in9b/1 -> Multiport Switch/3

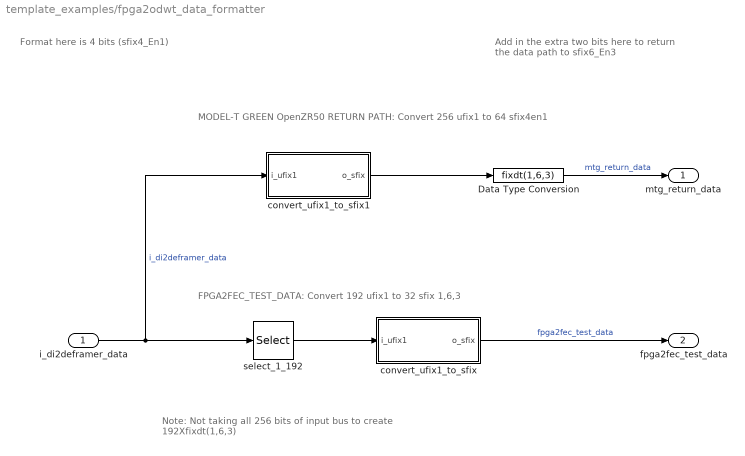
== system template_examples/fpga2odwt_data_formatter ==
  note: Format here is 4 bits (sfix4_En1)
  note: Add in the extra two bits here to return the data path to sfix6_En3
  note: Note:
      | Not taking all 256 bits of input bus to create 192Xfixdt(1,6,3)
  note: FPGA2FEC_TEST_DATA: Convert 192 ufix1 to 32 sfix 1,6,3
  note: MODEL-T GREEN OpenZR50 RETURN PATH: Convert 256 ufix1 to 64 sfix4en1
  i_di2deframer_data : Inport
  Data Type Conversion : DataTypeConversion  OutDataTypeStr=fixdt(1,6,3)  SaturateOnIntegerOverflow=off  RndMeth=Floor
  convert_ufix1_to_sfix : Subsystem  TreatAsAtomicUnit=on
  convert_ufix1_to_sfix1 : Subsystem  TreatAsAtomicUnit=on
  select_1_192 : Selector  InputPortWidth=256  IndexOptions=Index vector (dialog)  Indices=[1:192]  OutputSizes=1
  mtg_return_data : Outport
  fpga2fec_test_data : Outport  Port=2
  wires:
  Data Type Conversion/1 -> mtg_return_data/1  "mtg_return_data"
  i_di2deframer_data/1 -> convert_ufix1_to_sfix1/1(i_ufix1), select_1_192/1  "i_di2deframer_data"
  select_1_192/1 -> convert_ufix1_to_sfix/1(i_ufix1)
  convert_ufix1_to_sfix/1(o_sfix) -> fpga2fec_test_data/1  "fpga2fec_test_data"
  convert_ufix1_to_sfix1/1(o_sfix) -> Data Type Conversion/1

== system template_examples/ex21_convert_signed_to_ufix_to_signed/convert_sfix_to_ufix1 ==
  note: need to flip the output order of words to bits, so just used a selector, use the "u(:)" to turn into column vector to concatentate
  i_sfix : Inport  Partition=on  PartitionDimension=1  PartitionWidth=1  PartitionOffset=0
  For Each : ForEach  DisableCoverage=on
  Reshape : Reshape
  Selector : Selector  IndexMode=Zero-based  InputPortWidth=4  IndexOptions=Index vector (dialog)  Indices=[3:-1:0]  OutputSizes=1
  Word to Bits : hdlsllib/Logic and Bit Operations/Word to Bits  maxWordLength=4  bitOrder=LSB first
  o_ufix : Outport  ConcatenationDimension=1
  wires:
  i_sfix/1 -> Word to Bits/1
  Word to Bits/1 -> Selector/1
  Selector/1 -> Reshape/1
  Reshape/1 -> o_ufix/1

== system template_examples/ex21_convert_signed_to_ufix_to_signed/convert_ufix1_to_sfix ==
  i_ufix1 : Inport  Partition=on  PartitionDimension=1  PartitionWidth=4  PartitionOffset=0
  Bits to Word : hdlsllib/Logic and Bit Operations/Bits to Word  bitOrder=LSB first  signedOutputValues=Unsigned
  For Each : ForEach  DisableCoverage=on
  convert_to_signed : DataTypeConversion  OutDataTypeStr=fixdt(1,4,1)  ConvertRealWorld=Stored Integer (SI)  SaturateOnIntegerOverflow=off  RndMeth=Floor
  o_sfix : Outport  ConcatenationDimension=1
  wires:
  i_ufix1/1 -> Bits to Word/1
  Bits to Word/1 -> convert_to_signed/1
  convert_to_signed/1 -> o_sfix/1

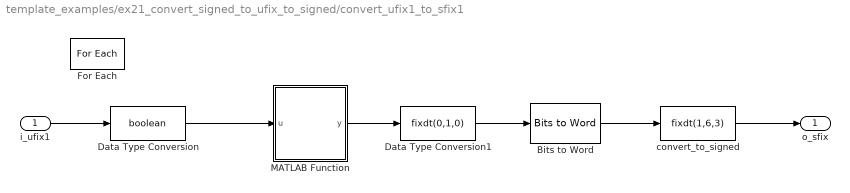
== system template_examples/ex21_convert_signed_to_ufix_to_signed/convert_ufix1_to_sfix1 ==
  i_ufix1 : Inport  Partition=on  PartitionDimension=1  PartitionWidth=6  PartitionOffset=0
  Bits to Word : hdlsllib/Logic and Bit Operations/Bits to Word
  Data Type Conversion : DataTypeConversion  OutDataTypeStr=boolean  SaturateOnIntegerOverflow=off  RndMeth=Floor
  Data Type Conversion1 : DataTypeConversion  OutDataTypeStr=fixdt(0,1,0)  SaturateOnIntegerOverflow=off  RndMeth=Floor
  For Each : ForEach  DisableCoverage=on
  MATLAB Function : MATLAB Function  TreatAsAtomicUnit=on
  convert_to_signed : DataTypeConversion  OutDataTypeStr=fixdt(1,6,3)  ConvertRealWorld=Stored Integer (SI)  SaturateOnIntegerOverflow=off  RndMeth=Floor
  o_sfix : Outport  ConcatenationDimension=1
  wires:
  i_ufix1/1 -> Data Type Conversion/1
  Data Type Conversion/1 -> MATLAB Function/1(u)
  convert_to_signed/1 -> o_sfix/1
  MATLAB Function/1(y) -> Data Type Conversion1/1
  Data Type Conversion1/1 -> Bits to Word/1
  Bits to Word/1 -> convert_to_signed/1

== system template_examples/fpga2odwt_data_formatter/convert_ufix1_to_sfix ==
  i_ufix1 : Inport  Partition=on  PartitionDimension=1  PartitionWidth=6  PartitionOffset=0
  Bits to Word : hdlsllib/Logic and Bit Operations/Bits to Word  bitOrder=LSB first  signedOutputValues=Unsigned
  For Each : ForEach  DisableCoverage=on
  convert_to_signed : DataTypeConversion  OutDataTypeStr=fixdt(1,6,3)  ConvertRealWorld=Stored Integer (SI)  SaturateOnIntegerOverflow=off  RndMeth=Floor
  o_sfix : Outport  ConcatenationDimension=1
  wires:
  convert_to_signed/1 -> o_sfix/1
  i_ufix1/1 -> Bits to Word/1
  Bits to Word/1 -> convert_to_signed/1

== system template_examples/fpga2odwt_data_formatter/convert_ufix1_to_sfix1 ==
  i_ufix1 : Inport  Partition=on  PartitionDimension=1  PartitionWidth=4  PartitionOffset=0
  Bits to Word : hdlsllib/Logic and Bit Operations/Bits to Word  bitOrder=LSB first  signedOutputValues=Unsigned
  For Each : ForEach  DisableCoverage=on
  convert_to_signed : DataTypeConversion  OutDataTypeStr=fixdt(1,4,1)  ConvertRealWorld=Stored Integer (SI)  SaturateOnIntegerOverflow=off  RndMeth=Floor
  o_sfix : Outport  ConcatenationDimension=1
  wires:
  convert_to_signed/1 -> o_sfix/1
  i_ufix1/1 -> Bits to Word/1
  Bits to Word/1 -> convert_to_signed/1

== matlab function template_examples/ex21_convert_signed_to_ufix_to_signed/convert_ufix1_to_sfix1/MATLAB Function ==
  data: u input; y output
function y = fcn(u)
y = flip(u);

== stateflow chart template_examples/ex11_fsms/ex11_moore_fsm_inherited_update_sf ==
  settings: sampleTime=1  stateMachineType=MOORE_MACHINE  executeAtInitialization=1
  state IDLE
    sm_out11a = true;
    sm_out11b = false;
  state ACTIVE2
    sm_out11a = false;
    sm_out11b = false;
  state ACTIVE1
    sm_out11a = true;
    sm_out11b = true;
  (default) -> IDLE
  ACTIVE2 -> IDLE : [sel11a]
  IDLE -> ACTIVE1 : [sel11a]
  ACTIVE1 -> ACTIVE2 : [sel11a]
  data: moore_fsm_ffMode output Enum: moore_fsm_ffModeType; sel11a input; sm_out11a output; sm_out11b output

== stateflow chart template_examples/ex11_fsms/ex11_moore_fsm_discrete_update_sf ==
  settings: updateMethod=DISCRETE  sampleTime=1  stateMachineType=MOORE_MACHINE  executeAtInitialization=1
  state IDLE
    sm_out11a = true;
    sm_out11b = false;
  state ACTIVE2
    sm_out11a = false;
    sm_out11b = false;
  state ACTIVE1
    sm_out11a = true;
    sm_out11b = true;
  (default) -> IDLE
  ACTIVE2 -> IDLE : [sel11a]
  IDLE -> ACTIVE1 : [sel11a]
  ACTIVE1 -> ACTIVE2 : [sel11a]
  data: moore_fsm_ffMode output Enum: moore_fsm_ffModeType; sel11a input; sm_out11a output; sm_out11b output

== matlab function template_examples/ex1b_data_enabled_ff/MATLAB Function ==
  data: vec_in1 input; u input; y output
function y = fcn(vec_in1, u)

y = uint8(vec_in1 & repmat(u,8,1));

== matlab function template_examples/ex11_fsms/ex11_moore_fsm_mf ==
  settings: fimath=|
      | fimath(...
      | 'RoundMode', 'nearest',...
      | 'OverflowMode', 'saturate',...
      | 'ProductMode', 'FullPrecision', 'ProductWordLength', 128,...
      | 'SumMode', 'FullPrecision', 'SumWordLength', 128,...
      | 'CastBeforeSum', true)
  data: sm_out11a output; sel11a input; sm_out11b output boolean size=1; mf_state output
function [sm_out11a, sm_out11b, mf_state] = fcn(sel11a)

persistent moore_state_reg;
if isempty(moore_state_reg)
    moore_state_reg = fi(0, 0, 2, 0);
end

IDLE = 0;
ACTIVE1 = 1;
ACTIVE2 = 2;

switch (moore_state_reg(1))

    case IDLE
        sm_out11a = true;
        sm_out11b = false;
        mf_state = moore_state_reg(1);

        if (~sel11a)
            moore_state_reg(1) = IDLE;
        else
            moore_state_reg(1) = ACTIVE1;
        end

    case ACTIVE1

        sm_out11a = true;
        sm_out11b = true;
        mf_state = moore_state_reg(1);

        if (~sel11a)
            moore_state_reg(1) = ACTIVE1;
        else
            moore_state_reg(1) = ACTIVE2;
        end

    case ACTIVE2
        sm_out11a = false;
        sm_out11b = false;
        mf_state = moore_state_reg(1);

        if (~sel11a)
            moore_state_reg(1) = ACTIVE2;
        else
            moore_state_reg(1) = IDLE;
        end

    otherwise
        mf_state = moore_state_reg(1);
        sm_out11a = false;
        sm_out11b = false;
end
